simulink model "Fourth_order_ODE"  (R2012b)
settings: Solver=ode23  StartTime=0.0  StopTime=2*pi  RelTol=1e-8
settings Model: Creator=David  LastModifiedBy=David

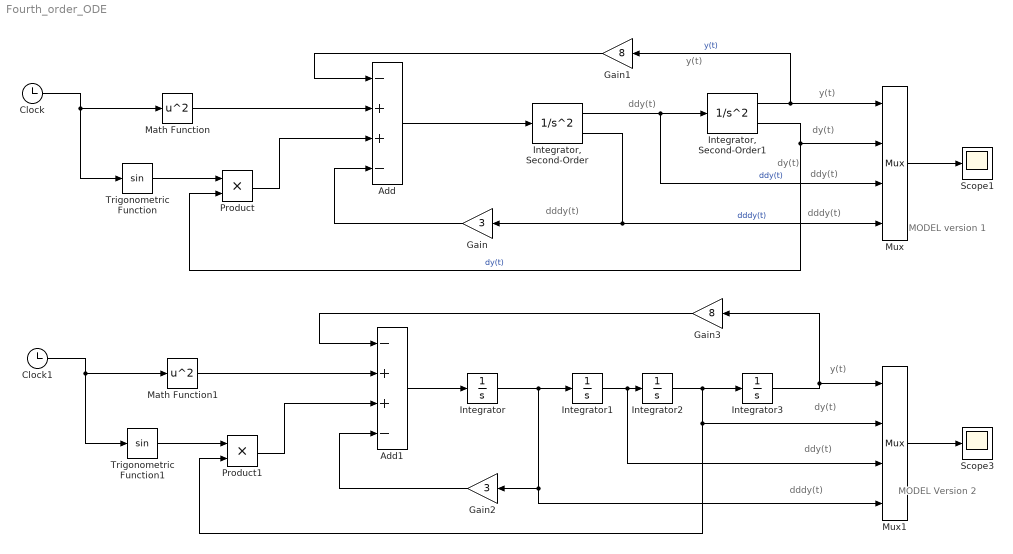
== system Fourth_order_ODE ==
  note: MODEL
      | Version 2
  note: MODEL
      | version 1
  note: dddy(t)
  note: ddy(t)
  note: dy(t)
  note: y(t)
  note: dddy(t)
  note: ddy(t)
  note: dy(t)
  note: dddy(t)
  note: ddy(t)
  note: dy(t)
  note: y(t)
  note: y(t)
  Add : Sum  Inputs=-++-
  Add1 : Sum  Inputs=-++-
  Clock : Clock
  Clock1 : Clock
  Gain : Gain  Gain=3
  Gain1 : Gain  Gain=8
  Gain2 : Gain  Gain=3
  Gain3 : Gain  Gain=8
  Integrator : Integrator  InitialCondition=5
  "Integrator, Second-Order" : SecondOrderIntegrator  ICX=11  ICDXDT=5
  "Integrator, Second-Order1" : SecondOrderIntegrator  ICX=50  ICDXDT=20
  Integrator1 : Integrator  InitialCondition=11
  Integrator2 : Integrator  InitialCondition=20
  Integrator3 : Integrator  InitialCondition=50
  Math Function : Math  Operator=square  SaturateOnIntegerOverflow=on
  Math Function1 : Math  Operator=square  SaturateOnIntegerOverflow=on
  Mux : Mux
  Mux1 : Mux
  Product : Product  RndMeth=Zero
  Product1 : Product  RndMeth=Zero
  Scope1 : Scope
      settings: ShowLegends=on
  Scope3 : Scope
      settings: SaveName=ScopeData3
  Trigonometric Function : Trigonometry
  Trigonometric Function1 : Trigonometry
  wires:
  Clock/1 -> Trigonometric Function/1, Math Function/1
  Add/1 -> "Integrator, Second-Order"/1
  "Integrator, Second-Order"/1 -> Mux/3, "Integrator, Second-Order1"/1  "ddy(t)"
  Gain/1 -> Add/4
  "Integrator, Second-Order1"/2 -> Product/2, Mux/2  "dy(t)"
  Trigonometric Function/1 -> Product/1
  Product/1 -> Add/3
  "Integrator, Second-Order1"/1 -> Mux/1, Gain1/1  "y(t)"
  Math Function/1 -> Add/2
  Gain1/1 -> Add/1
  "Integrator, Second-Order"/2 -> Gain/1, Mux/4  "dddy(t)"
  Mux/1 -> Scope1/1
  Clock1/1 -> Trigonometric Function1/1, Math Function1/1
  Add1/1 -> Integrator/1
  Gain2/1 -> Add1/4
  Trigonometric Function1/1 -> Product1/1
  Product1/1 -> Add1/3
  Math Function1/1 -> Add1/2
  Gain3/1 -> Add1/1
  Mux1/1 -> Scope3/1
  Integrator3/1 -> Gain3/1, Mux1/1
  Integrator2/1 -> Product1/2, Mux1/2, Integrator3/1
  Integrator/1 -> Mux1/4, Gain2/1, Integrator1/1
  Integrator1/1 -> Mux1/3, Integrator2/1
